simulink model "crazyDampedAngleSimu"  (R2015a)
settings: Solver=ode3  StartTime=0.0  StopTime=30  FixedStep=.01  RelTol=1e-3
values from neighbouring files (symbols this model uses):
  s = tf('s')    [ekstranul.m]
undefined symbols (not defined in the file or in its folder): Grx, rrx
libraries: cstblocks x7
settings Model: Creator=morten  LastModifiedBy=morten

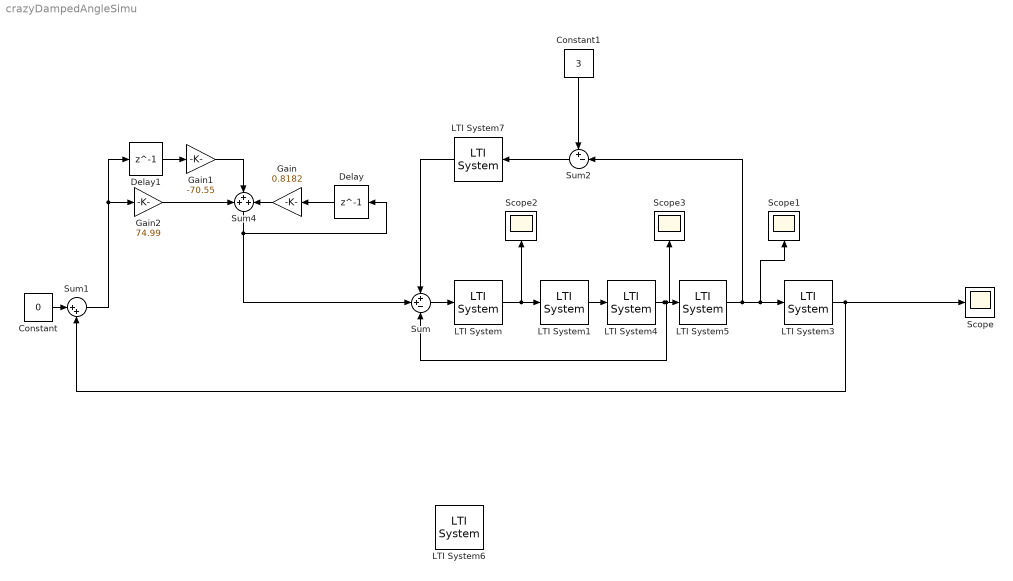
== system crazyDampedAngleSimu ==
  Constant : Constant  Value=0
  Constant1 : Constant  Value=3
  Delay : Delay  DelayLength=1
  Delay1 : Delay  DelayLength=1
  Gain : Gain  Gain=0.8182
  Gain1 : Gain  Gain=-70.55
  Gain2 : Gain  Gain=74.99
  LTI System : cstblocks/LTI System  sys=C1  IC=[]
  LTI System1 : cstblocks/LTI System  sys=Mx  IC=[]
  LTI System3 : cstblocks/LTI System  sys=W  IC=[]
  LTI System4 : cstblocks/LTI System  sys=Grx*rrx  IC=[]
  LTI System5 : cstblocks/LTI System  sys=1/s  IC=[]
  LTI System6 : cstblocks/LTI System  sys=C2  IC=[]
  LTI System7 : cstblocks/LTI System  sys=C3  IC=[]
  Scope{,1..3} (4 alike) : Scope
      Scope settings: YMin=-1  YMax=1
      Scope2 settings: SaveName=ScopeData2
      Scope3 settings: SaveName=ScopeData3
  Sum : Sum  Inputs=++-
  Sum1 : Sum  Inputs=|++
  Sum2 : Sum  Inputs=+-|
  Sum4 : Sum  Inputs=+++
  wires:
  LTI System1/1 -> LTI System4/1
  LTI System5/1 -> Sum2/2, Scope1/1, LTI System3/1
  LTI System4/1 -> Scope3/1, Sum/3, LTI System5/1
  Sum/1 -> LTI System/1
  Sum1/1 -> Gain2/1, Delay1/1
  Gain1/1 -> Sum4/2
  LTI System3/1 -> Sum1/2, Scope/1
  LTI System/1 -> LTI System1/1, Scope2/1
  Constant/1 -> Sum1/1
  Delay1/1 -> Gain1/1
  Delay/1 -> Gain/1
  Gain2/1 -> Sum4/1
  Sum4/1 -> Sum/2, Delay/1
  Gain/1 -> Sum4/3
  LTI System7/1 -> Sum/1
  Constant1/1 -> Sum2/1
  Sum2/1 -> LTI System7/1
